simulink model "TST_CrCtl_Governor"  (R2016b)
settings: Solver=FixedStepDiscrete  StartTime=0.0  StopTime=simTime  FixedStep=sampleTime  RelTol=1e-3
values from neighbouring files (symbols this model uses):
  testCase = 1    [initTST_CrCtl_Governor_001.m]    (also in initTST_CrCtl_Governor_002.m = 2; initTST_CrCtl_Governor_003.m = 3; initTST_CrCtl_Governor_004.m = 4; initTST_CrCtl_Governor_005.m = 5)
libraries: simulink x144, UnitTest_Lib x110
(part 4 of 7)

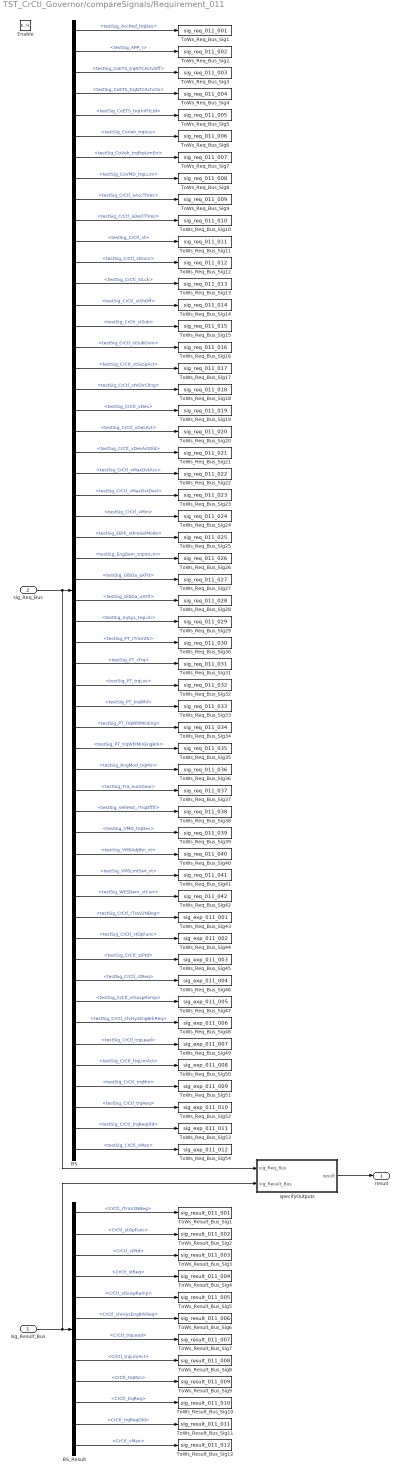
== system TST_CrCtl_Governor/compareSignals/Requirement_011 ==
  sig_Result_Bus : Inport
  sig_Req_Bus : Inport  Port=2
  Enable : EnablePort
  BS : BusSelector  OutputSignals=testSig_AccPed_trqDes,testSig_APP_r,testSig_CoETS_trqNTCActvOff,testSig_CoETS_trqNTCActvOn,testSig_CoETS_trqUnFltLtd,testSig_CoVeh_trqAcs,testSig_CoVeh_trqPrpLimErr,testSig_CoVMD_trqLLim,testSig_CrCtl_aAccThres,testSig_CrCtl_aDeclThres,testSig_CrCtl_st,testSig_CrCtl_stGvnr,testSig_CrCtl_stLck,testSig_CrCtl_stShOff,testSig_CrCtl_stSub,testSig_CrCtl_stSubGvnr,testSig_CrCtl_stSuspAct,testSig_CrCtl_stVDirChng,testSig_CrCtl_vDes,testSig_CrCtl_vDesAct,testSig_CrCtl_vDesActOld,testSig_CrCtl_vMaxDvtAcc,testSig_CrCtl_vMaxDvtDecl,testSig_CrCtl_vMin,testSig_EBrk_stPreSelMode,testSig_EngDem_trqInrLim,testSig_GlbDa_aXFlt,testSig_GlbDa_vXFlt,testSig_InjSys_trqLim,testSig_PT_rTraV2N,testSig_PT_rTrq,testSig_PT_trqLos,testSig_PT_trqWhl,testSig_PT_trqWhlMinEng,testSig_PT_trqWhlMinEngBrk,testSig_RngMod_trqMin,testSig_Tra_numGear,testSig_VehMot_rTrqDfftl,testSig_VMD_trqDes,testSig_VMSAdjBtn_st,testSig_VMSLmtSwt_st,testSig_WESDem_stCurr,testSig_CrCtl_rTraV2NBeg,testSig_CrCtl_stOpFunc,testSig_CrCtl_stPtd,testSig_CrCtl_stReq,testSig_CrCtl_stSuspRamp,testSig_CrCtl_stvHysEngBrkReq,testSig_CrCtl_trqLead,testSig_CrCtl_trqLimAct,testSig_CrCtl_trqMin,testSig_CrCtl_trqReq,testSig_CrCtl_trqReqOld,testSig_CrCtl_vMax
  BS_Result : BusSelector  OutputSignals=CrCtl_rTraV2NBeg,CrCtl_stOpFunc,CrCtl_stPtd,CrCtl_stReq,CrCtl_stSuspRamp,CrCtl_stvHysEngBrkReq,CrCtl_trqLead,CrCtl_trqLimAct,CrCtl_trqMin,CrCtl_trqReq,CrCtl_trqReqOld,CrCtl_vMax
  ToWs_Req_Bus_Sig1 : ToWorkspace  VariableName=sig_req_011_001  SaveFormat=Structure With Time
  ToWs_Req_Bus_Sig10 : ToWorkspace  VariableName=sig_req_011_010  SaveFormat=Structure With Time
  ToWs_Req_Bus_Sig11 : ToWorkspace  VariableName=sig_req_011_011  SaveFormat=Structure With Time
  ToWs_Req_Bus_Sig12 : ToWorkspace  VariableName=sig_req_011_012  SaveFormat=Structure With Time
  ToWs_Req_Bus_Sig13 : ToWorkspace  VariableName=sig_req_011_013  SaveFormat=Structure With Time
  ToWs_Req_Bus_Sig14 : ToWorkspace  VariableName=sig_req_011_014  SaveFormat=Structure With Time
  ToWs_Req_Bus_Sig15 : ToWorkspace  VariableName=sig_req_011_015  SaveFormat=Structure With Time
  ToWs_Req_Bus_Sig16 : ToWorkspace  VariableName=sig_req_011_016  SaveFormat=Structure With Time
  ToWs_Req_Bus_Sig17 : ToWorkspace  VariableName=sig_req_011_017  SaveFormat=Structure With Time
  ToWs_Req_Bus_Sig18 : ToWorkspace  VariableName=sig_req_011_018  SaveFormat=Structure With Time
  ToWs_Req_Bus_Sig19 : ToWorkspace  VariableName=sig_req_011_019  SaveFormat=Structure With Time
  ToWs_Req_Bus_Sig2 : ToWorkspace  VariableName=sig_req_011_002  SaveFormat=Structure With Time
  ToWs_Req_Bus_Sig20 : ToWorkspace  VariableName=sig_req_011_020  SaveFormat=Structure With Time
  ToWs_Req_Bus_Sig21 : ToWorkspace  VariableName=sig_req_011_021  SaveFormat=Structure With Time
  ToWs_Req_Bus_Sig22 : ToWorkspace  VariableName=sig_req_011_022  SaveFormat=Structure With Time
  ToWs_Req_Bus_Sig23 : ToWorkspace  VariableName=sig_req_011_023  SaveFormat=Structure With Time
  ToWs_Req_Bus_Sig24 : ToWorkspace  VariableName=sig_req_011_024  SaveFormat=Structure With Time
  ToWs_Req_Bus_Sig25 : ToWorkspace  VariableName=sig_req_011_025  SaveFormat=Structure With Time
  ToWs_Req_Bus_Sig26 : ToWorkspace  VariableName=sig_req_011_026  SaveFormat=Structure With Time
  ToWs_Req_Bus_Sig27 : ToWorkspace  VariableName=sig_req_011_027  SaveFormat=Structure With Time
  ToWs_Req_Bus_Sig28 : ToWorkspace  VariableName=sig_req_011_028  SaveFormat=Structure With Time
  ToWs_Req_Bus_Sig29 : ToWorkspace  VariableName=sig_req_011_029  SaveFormat=Structure With Time
  ToWs_Req_Bus_Sig3 : ToWorkspace  VariableName=sig_req_011_003  SaveFormat=Structure With Time
  ToWs_Req_Bus_Sig30 : ToWorkspace  VariableName=sig_req_011_030  SaveFormat=Structure With Time
  ToWs_Req_Bus_Sig31 : ToWorkspace  VariableName=sig_req_011_031  SaveFormat=Structure With Time
  ToWs_Req_Bus_Sig32 : ToWorkspace  VariableName=sig_req_011_032  SaveFormat=Structure With Time
  ToWs_Req_Bus_Sig33 : ToWorkspace  VariableName=sig_req_011_033  SaveFormat=Structure With Time
  ToWs_Req_Bus_Sig34 : ToWorkspace  VariableName=sig_req_011_034  SaveFormat=Structure With Time
  ToWs_Req_Bus_Sig35 : ToWorkspace  VariableName=sig_req_011_035  SaveFormat=Structure With Time
  ToWs_Req_Bus_Sig36 : ToWorkspace  VariableName=sig_req_011_036  SaveFormat=Structure With Time
  ToWs_Req_Bus_Sig37 : ToWorkspace  VariableName=sig_req_011_037  SaveFormat=Structure With Time
  ToWs_Req_Bus_Sig38 : ToWorkspace  VariableName=sig_req_011_038  SaveFormat=Structure With Time
  ToWs_Req_Bus_Sig39 : ToWorkspace  VariableName=sig_req_011_039  SaveFormat=Structure With Time
  ToWs_Req_Bus_Sig4 : ToWorkspace  VariableName=sig_req_011_004  SaveFormat=Structure With Time
  ToWs_Req_Bus_Sig40 : ToWorkspace  VariableName=sig_req_011_040  SaveFormat=Structure With Time
  ToWs_Req_Bus_Sig41 : ToWorkspace  VariableName=sig_req_011_041  SaveFormat=Structure With Time
  ToWs_Req_Bus_Sig42 : ToWorkspace  VariableName=sig_req_011_042  SaveFormat=Structure With Time
  ToWs_Req_Bus_Sig43 : ToWorkspace  VariableName=sig_exp_011_001  SaveFormat=Structure With Time
  ToWs_Req_Bus_Sig44 : ToWorkspace  VariableName=sig_exp_011_002  SaveFormat=Structure With Time
  ToWs_Req_Bus_Sig45 : ToWorkspace  VariableName=sig_exp_011_003  SaveFormat=Structure With Time
  ToWs_Req_Bus_Sig46 : ToWorkspace  VariableName=sig_exp_011_004  SaveFormat=Structure With Time
  ToWs_Req_Bus_Sig47 : ToWorkspace  VariableName=sig_exp_011_005  SaveFormat=Structure With Time
  ToWs_Req_Bus_Sig48 : ToWorkspace  VariableName=sig_exp_011_006  SaveFormat=Structure With Time
  ToWs_Req_Bus_Sig49 : ToWorkspace  VariableName=sig_exp_011_007  SaveFormat=Structure With Time
  ToWs_Req_Bus_Sig5 : ToWorkspace  VariableName=sig_req_011_005  SaveFormat=Structure With Time
  ToWs_Req_Bus_Sig50 : ToWorkspace  VariableName=sig_exp_011_008  SaveFormat=Structure With Time
  ToWs_Req_Bus_Sig51 : ToWorkspace  VariableName=sig_exp_011_009  SaveFormat=Structure With Time
  ToWs_Req_Bus_Sig52 : ToWorkspace  VariableName=sig_exp_011_010  SaveFormat=Structure With Time
  ToWs_Req_Bus_Sig53 : ToWorkspace  VariableName=sig_exp_011_011  SaveFormat=Structure With Time
  ToWs_Req_Bus_Sig54 : ToWorkspace  VariableName=sig_exp_011_012  SaveFormat=Structure With Time
  ToWs_Req_Bus_Sig6 : ToWorkspace  VariableName=sig_req_011_006  SaveFormat=Structure With Time
  ToWs_Req_Bus_Sig7 : ToWorkspace  VariableName=sig_req_011_007  SaveFormat=Structure With Time
  ToWs_Req_Bus_Sig8 : ToWorkspace  VariableName=sig_req_011_008  SaveFormat=Structure With Time
  ToWs_Req_Bus_Sig9 : ToWorkspace  VariableName=sig_req_011_009  SaveFormat=Structure With Time
  ToWs_Result_Bus_Sig1 : ToWorkspace  VariableName=sig_result_011_001  SaveFormat=Structure With Time
  ToWs_Result_Bus_Sig10 : ToWorkspace  VariableName=sig_result_011_010  SaveFormat=Structure With Time
  ToWs_Result_Bus_Sig11 : ToWorkspace  VariableName=sig_result_011_011  SaveFormat=Structure With Time
  ToWs_Result_Bus_Sig12 : ToWorkspace  VariableName=sig_result_011_012  SaveFormat=Structure With Time
  ToWs_Result_Bus_Sig2 : ToWorkspace  VariableName=sig_result_011_002  SaveFormat=Structure With Time
  ToWs_Result_Bus_Sig3 : ToWorkspace  VariableName=sig_result_011_003  SaveFormat=Structure With Time
  ToWs_Result_Bus_Sig4 : ToWorkspace  VariableName=sig_result_011_004  SaveFormat=Structure With Time
  ToWs_Result_Bus_Sig5 : ToWorkspace  VariableName=sig_result_011_005  SaveFormat=Structure With Time
  ToWs_Result_Bus_Sig6 : ToWorkspace  VariableName=sig_result_011_006  SaveFormat=Structure With Time
  ToWs_Result_Bus_Sig7 : ToWorkspace  VariableName=sig_result_011_007  SaveFormat=Structure With Time
  ToWs_Result_Bus_Sig8 : ToWorkspace  VariableName=sig_result_011_008  SaveFormat=Structure With Time
  ToWs_Result_Bus_Sig9 : ToWorkspace  VariableName=sig_result_011_009  SaveFormat=Structure With Time
  specifyOutputs : Subsystem
  result : Outport
  wires:
  sig_Req_Bus/1 -> BS/1, specifyOutputs/1(sig_Req_Bus)
  BS/1 -> ToWs_Req_Bus_Sig1/1  "<testSig_AccPed_trqDes>"
  BS/2 -> ToWs_Req_Bus_Sig2/1  "<testSig_APP_r>"
  BS/3 -> ToWs_Req_Bus_Sig3/1  "<testSig_CoETS_trqNTCActvOff>"
  BS/4 -> ToWs_Req_Bus_Sig4/1  "<testSig_CoETS_trqNTCActvOn>"
  BS/5 -> ToWs_Req_Bus_Sig5/1  "<testSig_CoETS_trqUnFltLtd>"
  BS/6 -> ToWs_Req_Bus_Sig6/1  "<testSig_CoVeh_trqAcs>"
  BS/7 -> ToWs_Req_Bus_Sig7/1  "<testSig_CoVeh_trqPrpLimErr>"
  BS/8 -> ToWs_Req_Bus_Sig8/1  "<testSig_CoVMD_trqLLim>"
  BS/9 -> ToWs_Req_Bus_Sig9/1  "<testSig_CrCtl_aAccThres>"
  BS/10 -> ToWs_Req_Bus_Sig10/1  "<testSig_CrCtl_aDeclThres>"
  BS/11 -> ToWs_Req_Bus_Sig11/1  "<testSig_CrCtl_st>"
  BS/12 -> ToWs_Req_Bus_Sig12/1  "<testSig_CrCtl_stGvnr>"
  BS/13 -> ToWs_Req_Bus_Sig13/1  "<testSig_CrCtl_stLck>"
  BS/14 -> ToWs_Req_Bus_Sig14/1  "<testSig_CrCtl_stShOff>"
  BS/15 -> ToWs_Req_Bus_Sig15/1  "<testSig_CrCtl_stSub>"
  BS/16 -> ToWs_Req_Bus_Sig16/1  "<testSig_CrCtl_stSubGvnr>"
  BS/17 -> ToWs_Req_Bus_Sig17/1  "<testSig_CrCtl_stSuspAct>"
  BS/18 -> ToWs_Req_Bus_Sig18/1  "<testSig_CrCtl_stVDirChng>"
  BS/19 -> ToWs_Req_Bus_Sig19/1  "<testSig_CrCtl_vDes>"
  BS/20 -> ToWs_Req_Bus_Sig20/1  "<testSig_CrCtl_vDesAct>"
  BS/21 -> ToWs_Req_Bus_Sig21/1  "<testSig_CrCtl_vDesActOld>"
  BS/22 -> ToWs_Req_Bus_Sig22/1  "<testSig_CrCtl_vMaxDvtAcc>"
  BS/23 -> ToWs_Req_Bus_Sig23/1  "<testSig_CrCtl_vMaxDvtDecl>"
  BS/24 -> ToWs_Req_Bus_Sig24/1  "<testSig_CrCtl_vMin>"
  BS/25 -> ToWs_Req_Bus_Sig25/1  "<testSig_EBrk_stPreSelMode>"
  BS/26 -> ToWs_Req_Bus_Sig26/1  "<testSig_EngDem_trqInrLim>"
  BS/27 -> ToWs_Req_Bus_Sig27/1  "<testSig_GlbDa_aXFlt>"
  BS/28 -> ToWs_Req_Bus_Sig28/1  "<testSig_GlbDa_vXFlt>"
  BS/29 -> ToWs_Req_Bus_Sig29/1  "<testSig_InjSys_trqLim>"
  BS/30 -> ToWs_Req_Bus_Sig30/1  "<testSig_PT_rTraV2N>"
  BS/31 -> ToWs_Req_Bus_Sig31/1  "<testSig_PT_rTrq>"
  BS/32 -> ToWs_Req_Bus_Sig32/1  "<testSig_PT_trqLos>"
  BS/33 -> ToWs_Req_Bus_Sig33/1  "<testSig_PT_trqWhl>"
  BS/34 -> ToWs_Req_Bus_Sig34/1  "<testSig_PT_trqWhlMinEng>"
  BS/35 -> ToWs_Req_Bus_Sig35/1  "<testSig_PT_trqWhlMinEngBrk>"
  BS/36 -> ToWs_Req_Bus_Sig36/1  "<testSig_RngMod_trqMin>"
  BS/37 -> ToWs_Req_Bus_Sig37/1  "<testSig_Tra_numGear>"
  BS/38 -> ToWs_Req_Bus_Sig38/1  "<testSig_VehMot_rTrqDfftl>"
  BS/39 -> ToWs_Req_Bus_Sig39/1  "<testSig_VMD_trqDes>"
  BS/40 -> ToWs_Req_Bus_Sig40/1  "<testSig_VMSAdjBtn_st>"
  BS/41 -> ToWs_Req_Bus_Sig41/1  "<testSig_VMSLmtSwt_st>"
  BS/42 -> ToWs_Req_Bus_Sig42/1  "<testSig_WESDem_stCurr>"
  BS/43 -> ToWs_Req_Bus_Sig43/1  "<testSig_CrCtl_rTraV2NBeg>"
  BS/44 -> ToWs_Req_Bus_Sig44/1  "<testSig_CrCtl_stOpFunc>"
  BS/45 -> ToWs_Req_Bus_Sig45/1  "<testSig_CrCtl_stPtd>"
  BS/46 -> ToWs_Req_Bus_Sig46/1  "<testSig_CrCtl_stReq>"
  BS/47 -> ToWs_Req_Bus_Sig47/1  "<testSig_CrCtl_stSuspRamp>"
  BS/48 -> ToWs_Req_Bus_Sig48/1  "<testSig_CrCtl_stvHysEngBrkReq>"
  BS/49 -> ToWs_Req_Bus_Sig49/1  "<testSig_CrCtl_trqLead>"
  BS/50 -> ToWs_Req_Bus_Sig50/1  "<testSig_CrCtl_trqLimAct>"
  BS/51 -> ToWs_Req_Bus_Sig51/1  "<testSig_CrCtl_trqMin>"
  BS/52 -> ToWs_Req_Bus_Sig52/1  "<testSig_CrCtl_trqReq>"
  BS/53 -> ToWs_Req_Bus_Sig53/1  "<testSig_CrCtl_trqReqOld>"
  BS/54 -> ToWs_Req_Bus_Sig54/1  "<testSig_CrCtl_vMax>"
  sig_Result_Bus/1 -> BS_Result/1, specifyOutputs/2(sig_Result_Bus)
  BS_Result/1 -> ToWs_Result_Bus_Sig1/1  "<CrCtl_rTraV2NBeg>"
  BS_Result/2 -> ToWs_Result_Bus_Sig2/1  "<CrCtl_stOpFunc>"
  BS_Result/3 -> ToWs_Result_Bus_Sig3/1  "<CrCtl_stPtd>"
  BS_Result/4 -> ToWs_Result_Bus_Sig4/1  "<CrCtl_stReq>"
  BS_Result/5 -> ToWs_Result_Bus_Sig5/1  "<CrCtl_stSuspRamp>"
  BS_Result/6 -> ToWs_Result_Bus_Sig6/1  "<CrCtl_stvHysEngBrkReq>"
  BS_Result/7 -> ToWs_Result_Bus_Sig7/1  "<CrCtl_trqLead>"
  BS_Result/8 -> ToWs_Result_Bus_Sig8/1  "<CrCtl_trqLimAct>"
  BS_Result/9 -> ToWs_Result_Bus_Sig9/1  "<CrCtl_trqMin>"
  BS_Result/10 -> ToWs_Result_Bus_Sig10/1  "<CrCtl_trqReq>"
  BS_Result/11 -> ToWs_Result_Bus_Sig11/1  "<CrCtl_trqReqOld>"
  BS_Result/12 -> ToWs_Result_Bus_Sig12/1  "<CrCtl_vMax>"
  specifyOutputs/1(result) -> result/1

== system TST_CrCtl_Governor/simulationInput/testSignals_R001 ==
  BC : BusCreator  Inputs=54
  spec_APP_r : FromWorkspace  VariableName=testSig_APP_r  Interpolate=off  OutputAfterFinalValue=Holding final value
  spec_AccPed_trqDes : FromWorkspace  VariableName=testSig_AccPed_trqDes  Interpolate=off  OutputAfterFinalValue=Holding final value
  spec_CoETS_trqNTCActvOff : FromWorkspace  VariableName=testSig_CoETS_trqNTCActvOff  Interpolate=off  OutputAfterFinalValue=Holding final value
  spec_CoETS_trqNTCActvOn : FromWorkspace  VariableName=testSig_CoETS_trqNTCActvOn  Interpolate=off  OutputAfterFinalValue=Holding final value
  spec_CoETS_trqUnFltLtd : FromWorkspace  VariableName=testSig_CoETS_trqUnFltLtd  Interpolate=off  OutputAfterFinalValue=Holding final value
  spec_CoVMD_trqLLim : FromWorkspace  VariableName=testSig_CoVMD_trqLLim  Interpolate=off  OutputAfterFinalValue=Holding final value
  spec_CoVeh_trqAcs : FromWorkspace  VariableName=testSig_CoVeh_trqAcs  Interpolate=off  OutputAfterFinalValue=Holding final value
  spec_CoVeh_trqPrpLimErr : FromWorkspace  VariableName=testSig_CoVeh_trqPrpLimErr  Interpolate=off  OutputAfterFinalValue=Holding final value
  spec_CrCtl_aAccThres : FromWorkspace  VariableName=testSig_CrCtl_aAccThres  Interpolate=off  OutputAfterFinalValue=Holding final value
  spec_CrCtl_aDeclThres : FromWorkspace  VariableName=testSig_CrCtl_aDeclThres  Interpolate=off  OutputAfterFinalValue=Holding final value
  spec_CrCtl_rTraV2NBeg : FromWorkspace  VariableName=testSig_CrCtl_rTraV2NBeg  Interpolate=off  OutputAfterFinalValue=Holding final value
  spec_CrCtl_st : FromWorkspace  VariableName=testSig_CrCtl_st  Interpolate=off  OutputAfterFinalValue=Holding final value
  spec_CrCtl_stGvnr : FromWorkspace  VariableName=testSig_CrCtl_stGvnr  Interpolate=off  OutputAfterFinalValue=Holding final value
  spec_CrCtl_stLck : FromWorkspace  VariableName=testSig_CrCtl_stLck  Interpolate=off  OutputAfterFinalValue=Holding final value
  spec_CrCtl_stOpFunc : FromWorkspace  VariableName=testSig_CrCtl_stOpFunc  Interpolate=off  OutputAfterFinalValue=Holding final value
  spec_CrCtl_stPtd : FromWorkspace  VariableName=testSig_CrCtl_stPtd  Interpolate=off  OutputAfterFinalValue=Holding final value
  spec_CrCtl_stReq : FromWorkspace  VariableName=testSig_CrCtl_stReq  Interpolate=off  OutputAfterFinalValue=Holding final value
  spec_CrCtl_stShOff : FromWorkspace  VariableName=testSig_CrCtl_stShOff  Interpolate=off  OutputAfterFinalValue=Holding final value
  spec_CrCtl_stSub : FromWorkspace  VariableName=testSig_CrCtl_stSub  Interpolate=off  OutputAfterFinalValue=Holding final value
  spec_CrCtl_stSubGvnr : FromWorkspace  VariableName=testSig_CrCtl_stSubGvnr  Interpolate=off  OutputAfterFinalValue=Holding final value
  spec_CrCtl_stSuspAct : FromWorkspace  VariableName=testSig_CrCtl_stSuspAct  Interpolate=off  OutputAfterFinalValue=Holding final value
  spec_CrCtl_stSuspRamp : FromWorkspace  VariableName=testSig_CrCtl_stSuspRamp  Interpolate=off  OutputAfterFinalValue=Holding final value
  spec_CrCtl_stVDirChng : FromWorkspace  VariableName=testSig_CrCtl_stVDirChng  Interpolate=off  OutputAfterFinalValue=Holding final value
  spec_CrCtl_stvHysEngBrkReq : FromWorkspace  VariableName=testSig_CrCtl_stvHysEngBrkReq  Interpolate=off  OutputAfterFinalValue=Holding final value
  spec_CrCtl_trqLead : FromWorkspace  VariableName=testSig_CrCtl_trqLead  Interpolate=off  OutputAfterFinalValue=Holding final value
  spec_CrCtl_trqLimAct : FromWorkspace  VariableName=testSig_CrCtl_trqLimAct  Interpolate=off  OutputAfterFinalValue=Holding final value
  spec_CrCtl_trqMin : FromWorkspace  VariableName=testSig_CrCtl_trqMin  Interpolate=off  OutputAfterFinalValue=Holding final value
  spec_CrCtl_trqReq : FromWorkspace  VariableName=testSig_CrCtl_trqReq  Interpolate=off  OutputAfterFinalValue=Holding final value
  spec_CrCtl_trqReqOld : FromWorkspace  VariableName=testSig_CrCtl_trqReqOld  Interpolate=off  OutputAfterFinalValue=Holding final value
  spec_CrCtl_vDes : FromWorkspace  VariableName=testSig_CrCtl_vDes  Interpolate=off  OutputAfterFinalValue=Holding final value
  spec_CrCtl_vDesAct : FromWorkspace  VariableName=testSig_CrCtl_vDesAct  Interpolate=off  OutputAfterFinalValue=Holding final value
  spec_CrCtl_vDesActOld : FromWorkspace  VariableName=testSig_CrCtl_vDesActOld  Interpolate=off  OutputAfterFinalValue=Holding final value
  spec_CrCtl_vMax : FromWorkspace  VariableName=testSig_CrCtl_vMax  Interpolate=off  OutputAfterFinalValue=Holding final value
  spec_CrCtl_vMaxDvtAcc : FromWorkspace  VariableName=testSig_CrCtl_vMaxDvtAcc  Interpolate=off  OutputAfterFinalValue=Holding final value
  spec_CrCtl_vMaxDvtDecl : FromWorkspace  VariableName=testSig_CrCtl_vMaxDvtDecl  Interpolate=off  OutputAfterFinalValue=Holding final value
  spec_CrCtl_vMin : FromWorkspace  VariableName=testSig_CrCtl_vMin  Interpolate=off  OutputAfterFinalValue=Holding final value
  spec_EBrk_stPreSelMode : FromWorkspace  VariableName=testSig_EBrk_stPreSelMode  Interpolate=off  OutputAfterFinalValue=Holding final value
  spec_EngDem_trqInrLim : FromWorkspace  VariableName=testSig_EngDem_trqInrLim  Interpolate=off  OutputAfterFinalValue=Holding final value
  spec_GlbDa_aXFlt : FromWorkspace  VariableName=testSig_GlbDa_aXFlt  Interpolate=off  OutputAfterFinalValue=Holding final value
  spec_GlbDa_vXFlt : FromWorkspace  VariableName=testSig_GlbDa_vXFlt  Interpolate=off  OutputAfterFinalValue=Holding final value
  spec_InjSys_trqLim : FromWorkspace  VariableName=testSig_InjSys_trqLim  Interpolate=off  OutputAfterFinalValue=Holding final value
  spec_PT_rTraV2N : FromWorkspace  VariableName=testSig_PT_rTraV2N  Interpolate=off  OutputAfterFinalValue=Holding final value
  spec_PT_rTrq : FromWorkspace  VariableName=testSig_PT_rTrq  Interpolate=off  OutputAfterFinalValue=Holding final value
  spec_PT_trqLos : FromWorkspace  VariableName=testSig_PT_trqLos  Interpolate=off  OutputAfterFinalValue=Holding final value
  spec_PT_trqWhl : FromWorkspace  VariableName=testSig_PT_trqWhl  Interpolate=off  OutputAfterFinalValue=Holding final value
  spec_PT_trqWhlMinEng : FromWorkspace  VariableName=testSig_PT_trqWhlMinEng  Interpolate=off  OutputAfterFinalValue=Holding final value
  spec_PT_trqWhlMinEngBrk : FromWorkspace  VariableName=testSig_PT_trqWhlMinEngBrk  Interpolate=off  OutputAfterFinalValue=Holding final value
  spec_RngMod_trqMin : FromWorkspace  VariableName=testSig_RngMod_trqMin  Interpolate=off  OutputAfterFinalValue=Holding final value
  spec_Tra_numGear : FromWorkspace  VariableName=testSig_Tra_numGear  Interpolate=off  OutputAfterFinalValue=Holding final value
  spec_VMD_trqDes : FromWorkspace  VariableName=testSig_VMD_trqDes  Interpolate=off  OutputAfterFinalValue=Holding final value
  spec_VMSAdjBtn_st : FromWorkspace  VariableName=testSig_VMSAdjBtn_st  Interpolate=off  OutputAfterFinalValue=Holding final value
  spec_VMSLmtSwt_st : FromWorkspace  VariableName=testSig_VMSLmtSwt_st  Interpolate=off  OutputAfterFinalValue=Holding final value
  spec_VehMot_rTrqDfftl : FromWorkspace  VariableName=testSig_VehMot_rTrqDfftl  Interpolate=off  OutputAfterFinalValue=Holding final value
  spec_WESDem_stCurr : FromWorkspace  VariableName=testSig_WESDem_stCurr  Interpolate=off  OutputAfterFinalValue=Holding final value
  testSignals : Outport
  wires:
  BC/1 -> testSignals/1
  spec_AccPed_trqDes/1 -> BC/1  "testSig_AccPed_trqDes"
  spec_APP_r/1 -> BC/2  "testSig_APP_r"
  spec_CoETS_trqNTCActvOff/1 -> BC/3  "testSig_CoETS_trqNTCActvOff"
  spec_CoETS_trqNTCActvOn/1 -> BC/4  "testSig_CoETS_trqNTCActvOn"
  spec_CoETS_trqUnFltLtd/1 -> BC/5  "testSig_CoETS_trqUnFltLtd"
  spec_CoVeh_trqAcs/1 -> BC/6  "testSig_CoVeh_trqAcs"
  spec_CoVeh_trqPrpLimErr/1 -> BC/7  "testSig_CoVeh_trqPrpLimErr"
  spec_CoVMD_trqLLim/1 -> BC/8  "testSig_CoVMD_trqLLim"
  spec_CrCtl_aAccThres/1 -> BC/9  "testSig_CrCtl_aAccThres"
  spec_CrCtl_aDeclThres/1 -> BC/10  "testSig_CrCtl_aDeclThres"
  spec_CrCtl_st/1 -> BC/11  "testSig_CrCtl_st"
  spec_CrCtl_stGvnr/1 -> BC/12  "testSig_CrCtl_stGvnr"
  spec_CrCtl_stLck/1 -> BC/13  "testSig_CrCtl_stLck"
  spec_CrCtl_stShOff/1 -> BC/14  "testSig_CrCtl_stShOff"
  spec_CrCtl_stSub/1 -> BC/15  "testSig_CrCtl_stSub"
  spec_CrCtl_stSubGvnr/1 -> BC/16  "testSig_CrCtl_stSubGvnr"
  spec_CrCtl_stSuspAct/1 -> BC/17  "testSig_CrCtl_stSuspAct"
  spec_CrCtl_stVDirChng/1 -> BC/18  "testSig_CrCtl_stVDirChng"
  spec_CrCtl_vDes/1 -> BC/19  "testSig_CrCtl_vDes"
  spec_CrCtl_vDesAct/1 -> BC/20  "testSig_CrCtl_vDesAct"
  spec_CrCtl_vDesActOld/1 -> BC/21  "testSig_CrCtl_vDesActOld"
  spec_CrCtl_vMaxDvtAcc/1 -> BC/22  "testSig_CrCtl_vMaxDvtAcc"
  spec_CrCtl_vMaxDvtDecl/1 -> BC/23  "testSig_CrCtl_vMaxDvtDecl"
  spec_CrCtl_vMin/1 -> BC/24  "testSig_CrCtl_vMin"
  spec_EBrk_stPreSelMode/1 -> BC/25  "testSig_EBrk_stPreSelMode"
  spec_EngDem_trqInrLim/1 -> BC/26  "testSig_EngDem_trqInrLim"
  spec_GlbDa_aXFlt/1 -> BC/27  "testSig_GlbDa_aXFlt"
  spec_GlbDa_vXFlt/1 -> BC/28  "testSig_GlbDa_vXFlt"
  spec_InjSys_trqLim/1 -> BC/29  "testSig_InjSys_trqLim"
  spec_PT_rTraV2N/1 -> BC/30  "testSig_PT_rTraV2N"
  spec_PT_rTrq/1 -> BC/31  "testSig_PT_rTrq"
  spec_PT_trqLos/1 -> BC/32  "testSig_PT_trqLos"
  spec_PT_trqWhl/1 -> BC/33  "testSig_PT_trqWhl"
  spec_PT_trqWhlMinEng/1 -> BC/34  "testSig_PT_trqWhlMinEng"
  spec_PT_trqWhlMinEngBrk/1 -> BC/35  "testSig_PT_trqWhlMinEngBrk"
  spec_RngMod_trqMin/1 -> BC/36  "testSig_RngMod_trqMin"
  spec_Tra_numGear/1 -> BC/37  "testSig_Tra_numGear"
  spec_VehMot_rTrqDfftl/1 -> BC/38  "testSig_VehMot_rTrqDfftl"
  spec_VMD_trqDes/1 -> BC/39  "testSig_VMD_trqDes"
  spec_VMSAdjBtn_st/1 -> BC/40  "testSig_VMSAdjBtn_st"
  spec_VMSLmtSwt_st/1 -> BC/41  "testSig_VMSLmtSwt_st"
  spec_WESDem_stCurr/1 -> BC/42  "testSig_WESDem_stCurr"
  spec_CrCtl_rTraV2NBeg/1 -> BC/43  "testSig_CrCtl_rTraV2NBeg"
  spec_CrCtl_stOpFunc/1 -> BC/44  "testSig_CrCtl_stOpFunc"
  spec_CrCtl_stPtd/1 -> BC/45  "testSig_CrCtl_stPtd"
  spec_CrCtl_stReq/1 -> BC/46  "testSig_CrCtl_stReq"
  spec_CrCtl_stSuspRamp/1 -> BC/47  "testSig_CrCtl_stSuspRamp"
  spec_CrCtl_stvHysEngBrkReq/1 -> BC/48  "testSig_CrCtl_stvHysEngBrkReq"
  spec_CrCtl_trqLead/1 -> BC/49  "testSig_CrCtl_trqLead"
  spec_CrCtl_trqLimAct/1 -> BC/50  "testSig_CrCtl_trqLimAct"
  spec_CrCtl_trqMin/1 -> BC/51  "testSig_CrCtl_trqMin"
  spec_CrCtl_trqReq/1 -> BC/52  "testSig_CrCtl_trqReq"
  spec_CrCtl_trqReqOld/1 -> BC/53  "testSig_CrCtl_trqReqOld"
  spec_CrCtl_vMax/1 -> BC/54  "testSig_CrCtl_vMax"

== system TST_CrCtl_Governor/simulationInput/testSignals_R002 ==
  BC : BusCreator  Inputs=54
  spec_APP_r : FromWorkspace  VariableName=testSig_APP_r  Interpolate=off  OutputAfterFinalValue=Holding final value
  spec_AccPed_trqDes : FromWorkspace  VariableName=testSig_AccPed_trqDes  Interpolate=off  OutputAfterFinalValue=Holding final value
  spec_CoETS_trqNTCActvOff : FromWorkspace  VariableName=testSig_CoETS_trqNTCActvOff  Interpolate=off  OutputAfterFinalValue=Holding final value
  spec_CoETS_trqNTCActvOn : FromWorkspace  VariableName=testSig_CoETS_trqNTCActvOn  Interpolate=off  OutputAfterFinalValue=Holding final value
  spec_CoETS_trqUnFltLtd : FromWorkspace  VariableName=testSig_CoETS_trqUnFltLtd  Interpolate=off  OutputAfterFinalValue=Holding final value
  spec_CoVMD_trqLLim : FromWorkspace  VariableName=testSig_CoVMD_trqLLim  Interpolate=off  OutputAfterFinalValue=Holding final value
  spec_CoVeh_trqAcs : FromWorkspace  VariableName=testSig_CoVeh_trqAcs  Interpolate=off  OutputAfterFinalValue=Holding final value
  spec_CoVeh_trqPrpLimErr : FromWorkspace  VariableName=testSig_CoVeh_trqPrpLimErr  Interpolate=off  OutputAfterFinalValue=Holding final value
  spec_CrCtl_aAccThres : FromWorkspace  VariableName=testSig_CrCtl_aAccThres  Interpolate=off  OutputAfterFinalValue=Holding final value
  spec_CrCtl_aDeclThres : FromWorkspace  VariableName=testSig_CrCtl_aDeclThres  Interpolate=off  OutputAfterFinalValue=Holding final value
  spec_CrCtl_rTraV2NBeg : FromWorkspace  VariableName=testSig_CrCtl_rTraV2NBeg  Interpolate=off  OutputAfterFinalValue=Holding final value
  spec_CrCtl_st : FromWorkspace  VariableName=testSig_CrCtl_st  Interpolate=off  OutputAfterFinalValue=Holding final value
  spec_CrCtl_stGvnr : FromWorkspace  VariableName=testSig_CrCtl_stGvnr  Interpolate=off  OutputAfterFinalValue=Holding final value
  spec_CrCtl_stLck : FromWorkspace  VariableName=testSig_CrCtl_stLck  Interpolate=off  OutputAfterFinalValue=Holding final value
  spec_CrCtl_stOpFunc : FromWorkspace  VariableName=testSig_CrCtl_stOpFunc  Interpolate=off  OutputAfterFinalValue=Holding final value
  spec_CrCtl_stPtd : FromWorkspace  VariableName=testSig_CrCtl_stPtd  Interpolate=off  OutputAfterFinalValue=Holding final value
  spec_CrCtl_stReq : FromWorkspace  VariableName=testSig_CrCtl_stReq  Interpolate=off  OutputAfterFinalValue=Holding final value
  spec_CrCtl_stShOff : FromWorkspace  VariableName=testSig_CrCtl_stShOff  Interpolate=off  OutputAfterFinalValue=Holding final value
  spec_CrCtl_stSub : FromWorkspace  VariableName=testSig_CrCtl_stSub  Interpolate=off  OutputAfterFinalValue=Holding final value
  spec_CrCtl_stSubGvnr : FromWorkspace  VariableName=testSig_CrCtl_stSubGvnr  Interpolate=off  OutputAfterFinalValue=Holding final value
  spec_CrCtl_stSuspAct : FromWorkspace  VariableName=testSig_CrCtl_stSuspAct  Interpolate=off  OutputAfterFinalValue=Holding final value
  spec_CrCtl_stSuspRamp : FromWorkspace  VariableName=testSig_CrCtl_stSuspRamp  Interpolate=off  OutputAfterFinalValue=Holding final value
  spec_CrCtl_stVDirChng : FromWorkspace  VariableName=testSig_CrCtl_stVDirChng  Interpolate=off  OutputAfterFinalValue=Holding final value
  spec_CrCtl_stvHysEngBrkReq : FromWorkspace  VariableName=testSig_CrCtl_stvHysEngBrkReq  Interpolate=off  OutputAfterFinalValue=Holding final value
  spec_CrCtl_trqLead : FromWorkspace  VariableName=testSig_CrCtl_trqLead  Interpolate=off  OutputAfterFinalValue=Holding final value
  spec_CrCtl_trqLimAct : FromWorkspace  VariableName=testSig_CrCtl_trqLimAct  Interpolate=off  OutputAfterFinalValue=Holding final value
  spec_CrCtl_trqMin : FromWorkspace  VariableName=testSig_CrCtl_trqMin  Interpolate=off  OutputAfterFinalValue=Holding final value
  spec_CrCtl_trqReq : FromWorkspace  VariableName=testSig_CrCtl_trqReq  Interpolate=off  OutputAfterFinalValue=Holding final value
  spec_CrCtl_trqReqOld : FromWorkspace  VariableName=testSig_CrCtl_trqReqOld  Interpolate=off  OutputAfterFinalValue=Holding final value
  spec_CrCtl_vDes : FromWorkspace  VariableName=testSig_CrCtl_vDes  Interpolate=off  OutputAfterFinalValue=Holding final value
  spec_CrCtl_vDesAct : FromWorkspace  VariableName=testSig_CrCtl_vDesAct  Interpolate=off  OutputAfterFinalValue=Holding final value
  spec_CrCtl_vDesActOld : FromWorkspace  VariableName=testSig_CrCtl_vDesActOld  Interpolate=off  OutputAfterFinalValue=Holding final value
  spec_CrCtl_vMax : FromWorkspace  VariableName=testSig_CrCtl_vMax  Interpolate=off  OutputAfterFinalValue=Holding final value
  spec_CrCtl_vMaxDvtAcc : FromWorkspace  VariableName=testSig_CrCtl_vMaxDvtAcc  Interpolate=off  OutputAfterFinalValue=Holding final value
  spec_CrCtl_vMaxDvtDecl : FromWorkspace  VariableName=testSig_CrCtl_vMaxDvtDecl  Interpolate=off  OutputAfterFinalValue=Holding final value
  spec_CrCtl_vMin : FromWorkspace  VariableName=testSig_CrCtl_vMin  Interpolate=off  OutputAfterFinalValue=Holding final value
  spec_EBrk_stPreSelMode : FromWorkspace  VariableName=testSig_EBrk_stPreSelMode  Interpolate=off  OutputAfterFinalValue=Holding final value
  spec_EngDem_trqInrLim : FromWorkspace  VariableName=testSig_EngDem_trqInrLim  Interpolate=off  OutputAfterFinalValue=Holding final value
  spec_GlbDa_aXFlt : FromWorkspace  VariableName=testSig_GlbDa_aXFlt  Interpolate=off  OutputAfterFinalValue=Holding final value
  spec_GlbDa_vXFlt : FromWorkspace  VariableName=testSig_GlbDa_vXFlt  Interpolate=off  OutputAfterFinalValue=Holding final value
  spec_InjSys_trqLim : FromWorkspace  VariableName=testSig_InjSys_trqLim  Interpolate=off  OutputAfterFinalValue=Holding final value
  spec_PT_rTraV2N : FromWorkspace  VariableName=testSig_PT_rTraV2N  Interpolate=off  OutputAfterFinalValue=Holding final value
  spec_PT_rTrq : FromWorkspace  VariableName=testSig_PT_rTrq  Interpolate=off  OutputAfterFinalValue=Holding final value
  spec_PT_trqLos : FromWorkspace  VariableName=testSig_PT_trqLos  Interpolate=off  OutputAfterFinalValue=Holding final value
  spec_PT_trqWhl : FromWorkspace  VariableName=testSig_PT_trqWhl  Interpolate=off  OutputAfterFinalValue=Holding final value
  spec_PT_trqWhlMinEng : FromWorkspace  VariableName=testSig_PT_trqWhlMinEng  Interpolate=off  OutputAfterFinalValue=Holding final value
  spec_PT_trqWhlMinEngBrk : FromWorkspace  VariableName=testSig_PT_trqWhlMinEngBrk  Interpolate=off  OutputAfterFinalValue=Holding final value
  spec_RngMod_trqMin : FromWorkspace  VariableName=testSig_RngMod_trqMin  Interpolate=off  OutputAfterFinalValue=Holding final value
  spec_Tra_numGear : FromWorkspace  VariableName=testSig_Tra_numGear  Interpolate=off  OutputAfterFinalValue=Holding final value
  spec_VMD_trqDes : FromWorkspace  VariableName=testSig_VMD_trqDes  Interpolate=off  OutputAfterFinalValue=Holding final value
  spec_VMSAdjBtn_st : FromWorkspace  VariableName=testSig_VMSAdjBtn_st  Interpolate=off  OutputAfterFinalValue=Holding final value
  spec_VMSLmtSwt_st : FromWorkspace  VariableName=testSig_VMSLmtSwt_st  Interpolate=off  OutputAfterFinalValue=Holding final value
  spec_VehMot_rTrqDfftl : FromWorkspace  VariableName=testSig_VehMot_rTrqDfftl  Interpolate=off  OutputAfterFinalValue=Holding final value
  spec_WESDem_stCurr : FromWorkspace  VariableName=testSig_WESDem_stCurr  Interpolate=off  OutputAfterFinalValue=Holding final value
  testSignals : Outport
  wires:
  BC/1 -> testSignals/1
  spec_AccPed_trqDes/1 -> BC/1  "testSig_AccPed_trqDes"
  spec_APP_r/1 -> BC/2  "testSig_APP_r"
  spec_CoETS_trqNTCActvOff/1 -> BC/3  "testSig_CoETS_trqNTCActvOff"
  spec_CoETS_trqNTCActvOn/1 -> BC/4  "testSig_CoETS_trqNTCActvOn"
  spec_CoETS_trqUnFltLtd/1 -> BC/5  "testSig_CoETS_trqUnFltLtd"
  spec_CoVeh_trqAcs/1 -> BC/6  "testSig_CoVeh_trqAcs"
  spec_CoVeh_trqPrpLimErr/1 -> BC/7  "testSig_CoVeh_trqPrpLimErr"
  spec_CoVMD_trqLLim/1 -> BC/8  "testSig_CoVMD_trqLLim"
  spec_CrCtl_aAccThres/1 -> BC/9  "testSig_CrCtl_aAccThres"
  spec_CrCtl_aDeclThres/1 -> BC/10  "testSig_CrCtl_aDeclThres"
  spec_CrCtl_st/1 -> BC/11  "testSig_CrCtl_st"
  spec_CrCtl_stGvnr/1 -> BC/12  "testSig_CrCtl_stGvnr"
  spec_CrCtl_stLck/1 -> BC/13  "testSig_CrCtl_stLck"
  spec_CrCtl_stShOff/1 -> BC/14  "testSig_CrCtl_stShOff"
  spec_CrCtl_stSub/1 -> BC/15  "testSig_CrCtl_stSub"
  spec_CrCtl_stSubGvnr/1 -> BC/16  "testSig_CrCtl_stSubGvnr"
  spec_CrCtl_stSuspAct/1 -> BC/17  "testSig_CrCtl_stSuspAct"
  spec_CrCtl_stVDirChng/1 -> BC/18  "testSig_CrCtl_stVDirChng"
  spec_CrCtl_vDes/1 -> BC/19  "testSig_CrCtl_vDes"
  spec_CrCtl_vDesAct/1 -> BC/20  "testSig_CrCtl_vDesAct"
  spec_CrCtl_vDesActOld/1 -> BC/21  "testSig_CrCtl_vDesActOld"
  spec_CrCtl_vMaxDvtAcc/1 -> BC/22  "testSig_CrCtl_vMaxDvtAcc"
  spec_CrCtl_vMaxDvtDecl/1 -> BC/23  "testSig_CrCtl_vMaxDvtDecl"
  spec_CrCtl_vMin/1 -> BC/24  "testSig_CrCtl_vMin"
  spec_EBrk_stPreSelMode/1 -> BC/25  "testSig_EBrk_stPreSelMode"
  spec_EngDem_trqInrLim/1 -> BC/26  "testSig_EngDem_trqInrLim"
  spec_GlbDa_aXFlt/1 -> BC/27  "testSig_GlbDa_aXFlt"
  spec_GlbDa_vXFlt/1 -> BC/28  "testSig_GlbDa_vXFlt"
  spec_InjSys_trqLim/1 -> BC/29  "testSig_InjSys_trqLim"
  spec_PT_rTraV2N/1 -> BC/30  "testSig_PT_rTraV2N"
  spec_PT_rTrq/1 -> BC/31  "testSig_PT_rTrq"
  spec_PT_trqLos/1 -> BC/32  "testSig_PT_trqLos"
  spec_PT_trqWhl/1 -> BC/33  "testSig_PT_trqWhl"
  spec_PT_trqWhlMinEng/1 -> BC/34  "testSig_PT_trqWhlMinEng"
  spec_PT_trqWhlMinEngBrk/1 -> BC/35  "testSig_PT_trqWhlMinEngBrk"
  spec_RngMod_trqMin/1 -> BC/36  "testSig_RngMod_trqMin"
  spec_Tra_numGear/1 -> BC/37  "testSig_Tra_numGear"
  spec_VehMot_rTrqDfftl/1 -> BC/38  "testSig_VehMot_rTrqDfftl"
  spec_VMD_trqDes/1 -> BC/39  "testSig_VMD_trqDes"
  spec_VMSAdjBtn_st/1 -> BC/40  "testSig_VMSAdjBtn_st"
  spec_VMSLmtSwt_st/1 -> BC/41  "testSig_VMSLmtSwt_st"
  spec_WESDem_stCurr/1 -> BC/42  "testSig_WESDem_stCurr"
  spec_CrCtl_rTraV2NBeg/1 -> BC/43  "testSig_CrCtl_rTraV2NBeg"
  spec_CrCtl_stOpFunc/1 -> BC/44  "testSig_CrCtl_stOpFunc"
  spec_CrCtl_stPtd/1 -> BC/45  "testSig_CrCtl_stPtd"
  spec_CrCtl_stReq/1 -> BC/46  "testSig_CrCtl_stReq"
  spec_CrCtl_stSuspRamp/1 -> BC/47  "testSig_CrCtl_stSuspRamp"
  spec_CrCtl_stvHysEngBrkReq/1 -> BC/48  "testSig_CrCtl_stvHysEngBrkReq"
  spec_CrCtl_trqLead/1 -> BC/49  "testSig_CrCtl_trqLead"
  spec_CrCtl_trqLimAct/1 -> BC/50  "testSig_CrCtl_trqLimAct"
  spec_CrCtl_trqMin/1 -> BC/51  "testSig_CrCtl_trqMin"
  spec_CrCtl_trqReq/1 -> BC/52  "testSig_CrCtl_trqReq"
  spec_CrCtl_trqReqOld/1 -> BC/53  "testSig_CrCtl_trqReqOld"
  spec_CrCtl_vMax/1 -> BC/54  "testSig_CrCtl_vMax"

== system TST_CrCtl_Governor/simulationInput/testSignals_R003 ==
  BC : BusCreator  Inputs=54
  spec_APP_r : FromWorkspace  VariableName=testSig_APP_r  Interpolate=off  OutputAfterFinalValue=Holding final value
  spec_AccPed_trqDes : FromWorkspace  VariableName=testSig_AccPed_trqDes  Interpolate=off  OutputAfterFinalValue=Holding final value
  spec_CoETS_trqNTCActvOff : FromWorkspace  VariableName=testSig_CoETS_trqNTCActvOff  Interpolate=off  OutputAfterFinalValue=Holding final value
  spec_CoETS_trqNTCActvOn : FromWorkspace  VariableName=testSig_CoETS_trqNTCActvOn  Interpolate=off  OutputAfterFinalValue=Holding final value
  spec_CoETS_trqUnFltLtd : FromWorkspace  VariableName=testSig_CoETS_trqUnFltLtd  Interpolate=off  OutputAfterFinalValue=Holding final value
  spec_CoVMD_trqLLim : FromWorkspace  VariableName=testSig_CoVMD_trqLLim  Interpolate=off  OutputAfterFinalValue=Holding final value
  spec_CoVeh_trqAcs : FromWorkspace  VariableName=testSig_CoVeh_trqAcs  Interpolate=off  OutputAfterFinalValue=Holding final value
  spec_CoVeh_trqPrpLimErr : FromWorkspace  VariableName=testSig_CoVeh_trqPrpLimErr  Interpolate=off  OutputAfterFinalValue=Holding final value
  spec_CrCtl_aAccThres : FromWorkspace  VariableName=testSig_CrCtl_aAccThres  Interpolate=off  OutputAfterFinalValue=Holding final value
  spec_CrCtl_aDeclThres : FromWorkspace  VariableName=testSig_CrCtl_aDeclThres  Interpolate=off  OutputAfterFinalValue=Holding final value
  spec_CrCtl_rTraV2NBeg : FromWorkspace  VariableName=testSig_CrCtl_rTraV2NBeg  Interpolate=off  OutputAfterFinalValue=Holding final value
  spec_CrCtl_st : FromWorkspace  VariableName=testSig_CrCtl_st  Interpolate=off  OutputAfterFinalValue=Holding final value
  spec_CrCtl_stGvnr : FromWorkspace  VariableName=testSig_CrCtl_stGvnr  Interpolate=off  OutputAfterFinalValue=Holding final value
  spec_CrCtl_stLck : FromWorkspace  VariableName=testSig_CrCtl_stLck  Interpolate=off  OutputAfterFinalValue=Holding final value
  spec_CrCtl_stOpFunc : FromWorkspace  VariableName=testSig_CrCtl_stOpFunc  Interpolate=off  OutputAfterFinalValue=Holding final value
  spec_CrCtl_stPtd : FromWorkspace  VariableName=testSig_CrCtl_stPtd  Interpolate=off  OutputAfterFinalValue=Holding final value
  spec_CrCtl_stReq : FromWorkspace  VariableName=testSig_CrCtl_stReq  Interpolate=off  OutputAfterFinalValue=Holding final value
  spec_CrCtl_stShOff : FromWorkspace  VariableName=testSig_CrCtl_stShOff  Interpolate=off  OutputAfterFinalValue=Holding final value
  spec_CrCtl_stSub : FromWorkspace  VariableName=testSig_CrCtl_stSub  Interpolate=off  OutputAfterFinalValue=Holding final value
  spec_CrCtl_stSubGvnr : FromWorkspace  VariableName=testSig_CrCtl_stSubGvnr  Interpolate=off  OutputAfterFinalValue=Holding final value
  spec_CrCtl_stSuspAct : FromWorkspace  VariableName=testSig_CrCtl_stSuspAct  Interpolate=off  OutputAfterFinalValue=Holding final value
  spec_CrCtl_stSuspRamp : FromWorkspace  VariableName=testSig_CrCtl_stSuspRamp  Interpolate=off  OutputAfterFinalValue=Holding final value
  spec_CrCtl_stVDirChng : FromWorkspace  VariableName=testSig_CrCtl_stVDirChng  Interpolate=off  OutputAfterFinalValue=Holding final value
  spec_CrCtl_stvHysEngBrkReq : FromWorkspace  VariableName=testSig_CrCtl_stvHysEngBrkReq  Interpolate=off  OutputAfterFinalValue=Holding final value
  spec_CrCtl_trqLead : FromWorkspace  VariableName=testSig_CrCtl_trqLead  Interpolate=off  OutputAfterFinalValue=Holding final value
  spec_CrCtl_trqLimAct : FromWorkspace  VariableName=testSig_CrCtl_trqLimAct  Interpolate=off  OutputAfterFinalValue=Holding final value
  spec_CrCtl_trqMin : FromWorkspace  VariableName=testSig_CrCtl_trqMin  Interpolate=off  OutputAfterFinalValue=Holding final value
  spec_CrCtl_trqReq : FromWorkspace  VariableName=testSig_CrCtl_trqReq  Interpolate=off  OutputAfterFinalValue=Holding final value
  spec_CrCtl_trqReqOld : FromWorkspace  VariableName=testSig_CrCtl_trqReqOld  Interpolate=off  OutputAfterFinalValue=Holding final value
  spec_CrCtl_vDes : FromWorkspace  VariableName=testSig_CrCtl_vDes  Interpolate=off  OutputAfterFinalValue=Holding final value
  spec_CrCtl_vDesAct : FromWorkspace  VariableName=testSig_CrCtl_vDesAct  Interpolate=off  OutputAfterFinalValue=Holding final value
  spec_CrCtl_vDesActOld : FromWorkspace  VariableName=testSig_CrCtl_vDesActOld  Interpolate=off  OutputAfterFinalValue=Holding final value
  spec_CrCtl_vMax : FromWorkspace  VariableName=testSig_CrCtl_vMax  Interpolate=off  OutputAfterFinalValue=Holding final value
  spec_CrCtl_vMaxDvtAcc : FromWorkspace  VariableName=testSig_CrCtl_vMaxDvtAcc  Interpolate=off  OutputAfterFinalValue=Holding final value
  spec_CrCtl_vMaxDvtDecl : FromWorkspace  VariableName=testSig_CrCtl_vMaxDvtDecl  Interpolate=off  OutputAfterFinalValue=Holding final value
  spec_CrCtl_vMin : FromWorkspace  VariableName=testSig_CrCtl_vMin  Interpolate=off  OutputAfterFinalValue=Holding final value
  spec_EBrk_stPreSelMode : FromWorkspace  VariableName=testSig_EBrk_stPreSelMode  Interpolate=off  OutputAfterFinalValue=Holding final value
  spec_EngDem_trqInrLim : FromWorkspace  VariableName=testSig_EngDem_trqInrLim  Interpolate=off  OutputAfterFinalValue=Holding final value
  spec_GlbDa_aXFlt : FromWorkspace  VariableName=testSig_GlbDa_aXFlt  Interpolate=off  OutputAfterFinalValue=Holding final value
  spec_GlbDa_vXFlt : FromWorkspace  VariableName=testSig_GlbDa_vXFlt  Interpolate=off  OutputAfterFinalValue=Holding final value
  spec_InjSys_trqLim : FromWorkspace  VariableName=testSig_InjSys_trqLim  Interpolate=off  OutputAfterFinalValue=Holding final value
  spec_PT_rTraV2N : FromWorkspace  VariableName=testSig_PT_rTraV2N  Interpolate=off  OutputAfterFinalValue=Holding final value
  spec_PT_rTrq : FromWorkspace  VariableName=testSig_PT_rTrq  Interpolate=off  OutputAfterFinalValue=Holding final value
  spec_PT_trqLos : FromWorkspace  VariableName=testSig_PT_trqLos  Interpolate=off  OutputAfterFinalValue=Holding final value
  spec_PT_trqWhl : FromWorkspace  VariableName=testSig_PT_trqWhl  Interpolate=off  OutputAfterFinalValue=Holding final value
  spec_PT_trqWhlMinEng : FromWorkspace  VariableName=testSig_PT_trqWhlMinEng  Interpolate=off  OutputAfterFinalValue=Holding final value
  spec_PT_trqWhlMinEngBrk : FromWorkspace  VariableName=testSig_PT_trqWhlMinEngBrk  Interpolate=off  OutputAfterFinalValue=Holding final value
  spec_RngMod_trqMin : FromWorkspace  VariableName=testSig_RngMod_trqMin  Interpolate=off  OutputAfterFinalValue=Holding final value
  spec_Tra_numGear : FromWorkspace  VariableName=testSig_Tra_numGear  Interpolate=off  OutputAfterFinalValue=Holding final value
  spec_VMD_trqDes : FromWorkspace  VariableName=testSig_VMD_trqDes  Interpolate=off  OutputAfterFinalValue=Holding final value
  spec_VMSAdjBtn_st : FromWorkspace  VariableName=testSig_VMSAdjBtn_st  Interpolate=off  OutputAfterFinalValue=Holding final value
  spec_VMSLmtSwt_st : FromWorkspace  VariableName=testSig_VMSLmtSwt_st  Interpolate=off  OutputAfterFinalValue=Holding final value
  spec_VehMot_rTrqDfftl : FromWorkspace  VariableName=testSig_VehMot_rTrqDfftl  Interpolate=off  OutputAfterFinalValue=Holding final value
  spec_WESDem_stCurr : FromWorkspace  VariableName=testSig_WESDem_stCurr  Interpolate=off  OutputAfterFinalValue=Holding final value
  testSignals : Outport
  wires:
  BC/1 -> testSignals/1
  spec_AccPed_trqDes/1 -> BC/1  "testSig_AccPed_trqDes"
  spec_APP_r/1 -> BC/2  "testSig_APP_r"
  spec_CoETS_trqNTCActvOff/1 -> BC/3  "testSig_CoETS_trqNTCActvOff"
  spec_CoETS_trqNTCActvOn/1 -> BC/4  "testSig_CoETS_trqNTCActvOn"
  spec_CoETS_trqUnFltLtd/1 -> BC/5  "testSig_CoETS_trqUnFltLtd"
  spec_CoVeh_trqAcs/1 -> BC/6  "testSig_CoVeh_trqAcs"
  spec_CoVeh_trqPrpLimErr/1 -> BC/7  "testSig_CoVeh_trqPrpLimErr"
  spec_CoVMD_trqLLim/1 -> BC/8  "testSig_CoVMD_trqLLim"
  spec_CrCtl_aAccThres/1 -> BC/9  "testSig_CrCtl_aAccThres"
  spec_CrCtl_aDeclThres/1 -> BC/10  "testSig_CrCtl_aDeclThres"
  spec_CrCtl_st/1 -> BC/11  "testSig_CrCtl_st"
  spec_CrCtl_stGvnr/1 -> BC/12  "testSig_CrCtl_stGvnr"
  spec_CrCtl_stLck/1 -> BC/13  "testSig_CrCtl_stLck"
  spec_CrCtl_stShOff/1 -> BC/14  "testSig_CrCtl_stShOff"
  spec_CrCtl_stSub/1 -> BC/15  "testSig_CrCtl_stSub"
  spec_CrCtl_stSubGvnr/1 -> BC/16  "testSig_CrCtl_stSubGvnr"
  spec_CrCtl_stSuspAct/1 -> BC/17  "testSig_CrCtl_stSuspAct"
  spec_CrCtl_stVDirChng/1 -> BC/18  "testSig_CrCtl_stVDirChng"
  spec_CrCtl_vDes/1 -> BC/19  "testSig_CrCtl_vDes"
  spec_CrCtl_vDesAct/1 -> BC/20  "testSig_CrCtl_vDesAct"
  spec_CrCtl_vDesActOld/1 -> BC/21  "testSig_CrCtl_vDesActOld"
  spec_CrCtl_vMaxDvtAcc/1 -> BC/22  "testSig_CrCtl_vMaxDvtAcc"
  spec_CrCtl_vMaxDvtDecl/1 -> BC/23  "testSig_CrCtl_vMaxDvtDecl"
  spec_CrCtl_vMin/1 -> BC/24  "testSig_CrCtl_vMin"
  spec_EBrk_stPreSelMode/1 -> BC/25  "testSig_EBrk_stPreSelMode"
  spec_EngDem_trqInrLim/1 -> BC/26  "testSig_EngDem_trqInrLim"
  spec_GlbDa_aXFlt/1 -> BC/27  "testSig_GlbDa_aXFlt"
  spec_GlbDa_vXFlt/1 -> BC/28  "testSig_GlbDa_vXFlt"
  spec_InjSys_trqLim/1 -> BC/29  "testSig_InjSys_trqLim"
  spec_PT_rTraV2N/1 -> BC/30  "testSig_PT_rTraV2N"
  spec_PT_rTrq/1 -> BC/31  "testSig_PT_rTrq"
  spec_PT_trqLos/1 -> BC/32  "testSig_PT_trqLos"
  spec_PT_trqWhl/1 -> BC/33  "testSig_PT_trqWhl"
  spec_PT_trqWhlMinEng/1 -> BC/34  "testSig_PT_trqWhlMinEng"
  spec_PT_trqWhlMinEngBrk/1 -> BC/35  "testSig_PT_trqWhlMinEngBrk"
  spec_RngMod_trqMin/1 -> BC/36  "testSig_RngMod_trqMin"
  spec_Tra_numGear/1 -> BC/37  "testSig_Tra_numGear"
  spec_VehMot_rTrqDfftl/1 -> BC/38  "testSig_VehMot_rTrqDfftl"
  spec_VMD_trqDes/1 -> BC/39  "testSig_VMD_trqDes"
  spec_VMSAdjBtn_st/1 -> BC/40  "testSig_VMSAdjBtn_st"
  spec_VMSLmtSwt_st/1 -> BC/41  "testSig_VMSLmtSwt_st"
  spec_WESDem_stCurr/1 -> BC/42  "testSig_WESDem_stCurr"
  spec_CrCtl_rTraV2NBeg/1 -> BC/43  "testSig_CrCtl_rTraV2NBeg"
  spec_CrCtl_stOpFunc/1 -> BC/44  "testSig_CrCtl_stOpFunc"
  spec_CrCtl_stPtd/1 -> BC/45  "testSig_CrCtl_stPtd"
  spec_CrCtl_stReq/1 -> BC/46  "testSig_CrCtl_stReq"
  spec_CrCtl_stSuspRamp/1 -> BC/47  "testSig_CrCtl_stSuspRamp"
  spec_CrCtl_stvHysEngBrkReq/1 -> BC/48  "testSig_CrCtl_stvHysEngBrkReq"
  spec_CrCtl_trqLead/1 -> BC/49  "testSig_CrCtl_trqLead"
  spec_CrCtl_trqLimAct/1 -> BC/50  "testSig_CrCtl_trqLimAct"
  spec_CrCtl_trqMin/1 -> BC/51  "testSig_CrCtl_trqMin"
  spec_CrCtl_trqReq/1 -> BC/52  "testSig_CrCtl_trqReq"
  spec_CrCtl_trqReqOld/1 -> BC/53  "testSig_CrCtl_trqReqOld"
  spec_CrCtl_vMax/1 -> BC/54  "testSig_CrCtl_vMax"
